simulink model "b6_goto_target"  (R2021b)
settings: Solver=VariableStepAuto  StartTime=0.0  StopTime=inf  FixedStep=0.0001  RelTol=1e-3
PreLoadFcn:
  | % Simulation parameters
  | %load exampleMap
  | 
  | % Lidar parameters
  | sensorOffset = [0,0];
  | scanAngles = linspace(-pi/3,pi/3,20)';%y = linspace(x1,x2,n) 生成 n 个点。这些点的间距为 (x2-x1)/(n-1)。
  | maxRange = 0.4;
InitFcn:
  | sampleTime = 0.05;
  | nMedianSize=3;
  |  %load boundaryMap
  | 
  | % Robot parameters
  | wheelRadius = 0.0303;
  | robotRadius = 0.06;   %小车在仿真中显示的圆形的半径大小
  | Trackwidth = 0.0847;  %定义向量场直方图算法中小车的宽度
  | 
  | % Lidar parameters
  | sensorOffset = [0,0];
  | scanAngles = linspace(-pi/3,pi/3,20)';%y = linspace(x1,x2,n) 生成 n 个点。这些点的间距为 (x2-x1)/(n-1)。
  | maxRange = 0.4;
  | 
  | %%%%%%
  | ks=1;
  | 
  | 
  | A=0.5;
  | C=1.5;
  | B=(A+C)/2;
  | 
  | wp1=[A,A; B,A;  C,A; C,B;C,C; B,C; A,C;A,B];
  | bainjie2=[-0.5,-0.5;2.5,-0.5;-0.5,2.5;2.5,2.5;]
  | WAY_P=[wp1;wp1;wp1;wp1];
  | Target=[wp1;bainjie2];
  | 
  | %%%%%%%%%%%%%%%%%%%%%%%%%%%%%%%%%%%%%%%
  | Target_robot_4=[A  A]
  | Target_robot_5=[B  A]
  | Target_robot_6=[C  A]
  | 
  | Target_robot_1=[C  C]
  | Target_robot_2=[B  C]
  | Target_robot_3=[A  C]
  | 
  | 
  | %%%%%%%%%%%%%%%%%%%%%%%%%%%%%%%%%%%%
  | 
  | 
  | init_pose_1=[A    A  pi/2]';
  | init_pose_2=[B    A  pi/2]';
  | init_pose_3=[C    A  pi/2]';
  | init_pose_4=[C    C  -pi/2]';
  | init_pose_5=[B    C  -pi/2]';
  | init_pose_6=[A    C  -pi/2]';
  | 
  | 
  | 
  | 
  | %{
  | %初始位置 交叉
  | 
  | init_pose_1=[C    C    0]';
  | init_pose_2=[B    C    0]';
  | init_pose_3=[A    C  0]';
  | init_pose_4=[A    A  0]';
  | init_pose_5=[B    A  0]';
  | init_pose_6=[C    A  0]';
  | 
  | 
  | 
  | 
  | 
  | %初始位置
  | 
  | init_pose_1=[1    1    0]';
  | init_pose_2=[1.8  1    0]';
  | init_pose_3=[0.4  1.8  0]';
  | init_pose_4=[1.6  1.6  0]';
  | init_pose_5=[0.4  0.8  0]';
  | init_pose_6=[0.8  0.6  0]';
  | %}
  | 
  | 
  | % paremeters of pure persuit
  | desired_v=0.2
  | desired_w=10
  | desired_lookahead=0.1
  | 
  | % paremeters of recovery
  | %recovery_w=0.5
  | recovery_w=2
undefined symbols (not defined in the file or in its folder): Angular, DiscIntNeverNeededParam, Linear, Pose, Twist
libraries: robotlib x45, dspstat3 x18, mobileRoboticsLib x13, robotalgslib x12, robotmobilelib x6
(part 1 of 4)
settings Model: SimulationMode=accelerator  Creator=scastro  LastModifiedBy=FCS
settings SolverCC: AlgebraicLoopSolver=TrustRegion
settings DataIOCC: ReturnWorkspaceOutputs=off
settings OptimizationCC: EnhancedBackFolding=on  PassReuseOutputArgsAs=Individual arguments  ZeroExternalMemoryAtStartup=off  ZeroInternalMemoryAtStartup=off  MaxStackSize=64  OptimizeBlockOrder=speed  DifferentSizesBufferReuse=on  OptimizationCustomize=off  EfficientTunableParamExpr=on
settings DebuggingCC: ParameterTunabilityLossMsg=error  PregeneratedLibrarySubsystemCodeDiagnostic=none  SFMachineParentedDataDiag=warning  ArithmeticOperatorsInVariantConditions=warning
settings HardwareCC: ProdBitPerPointer=32  ProdBitPerSizeT=32  ProdBitPerPtrDiffT=32  ProdLargestAtomicFloat=None  ProdIntDivRoundTo=Undefined  ProdEndianess=Unspecified  ProdWordSize=32  ProdHWDeviceType=Generic->Unspecified (assume 32-bit Generic)
settings SFSimCC: SimUseLocalCustomCode=off  CustomCodeUndefinedFunction=UseInterfaceOnly
settings RTWCC: Description=Embedded Coder  SystemTargetFile=ert.tlc  HardwareBoard=Robot Operating System (ROS)  TLCOptions="-aInlineSetEventsForThisBaseRateFcn=TLC_FALSE -aSuppressMultiTaskScheduler=TLC_FALSE  -aRateBasedStepFcn=0"  TemplateMakefile=ert_default_tmf  RTWUseLocalCustomCode=off  Toolchain=Catkin  TargetLang=C++
settings CodeAppCC: ForceParamTrailComments=on  IgnoreCustomStorageClasses=off  OperatorAnnotations=on  SimulinkDataObjDesc=on  SFDataObjDesc=on  InsertBlockDesc=on

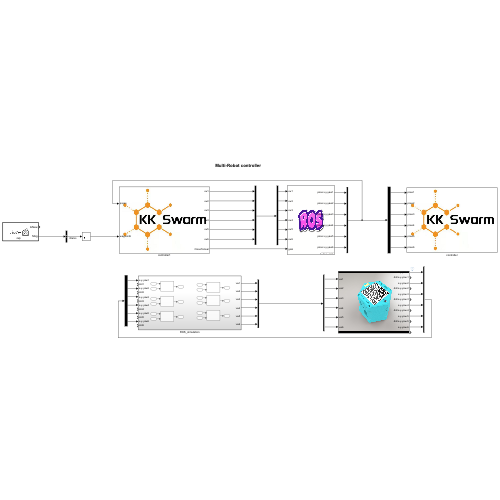
[thumbnail: Simulink's stored preview of the top-level diagram]
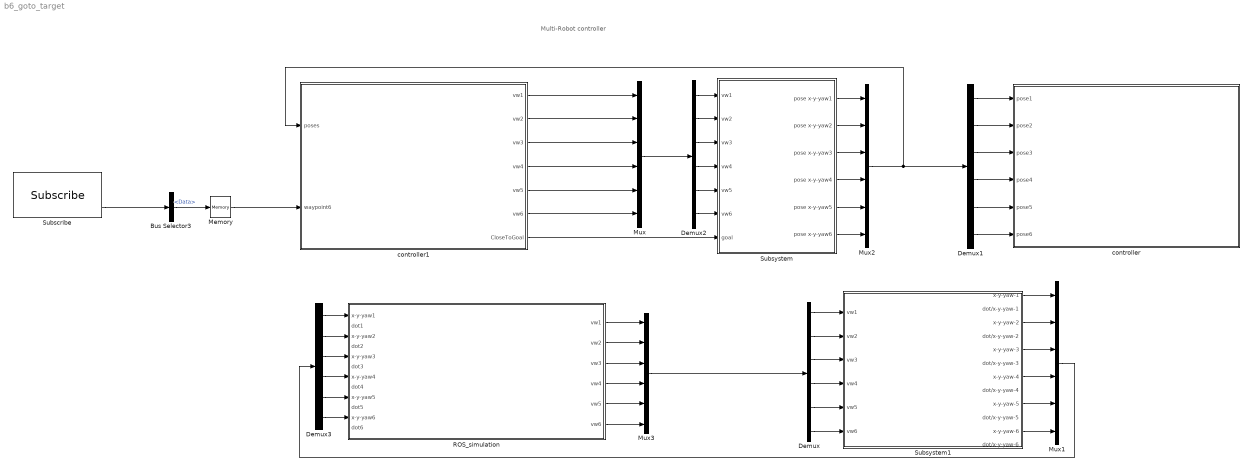
== system b6_goto_target ==
  note: Multi-Robot controller
  Bus Selector3 : BusSelector  OutputSignals=Data
  Demux{,1..3} (4 alike) : Demux  Outputs=6
  Memory : Memory  InitialCondition=123567
  Mux{,1..3} (4 alike) : Mux  Inputs=6
  ROS_simulation : Subsystem
  Subscribe : robotlib/Subscribe  topicSource=Select from ROS network  topic=/wp  messageType=std_msgs/Float64  SampleTime=-1  legacyBusStruct=off  messageQueueLength=51
  Subsystem : Subsystem
      mask Display: image('$imagefile'); % 使用工具条上的 "编辑图像" 进行更改。
  Subsystem1 : Subsystem
      mask Display: image('$imagefile'); % 使用工具条上的 "编辑图像" 进行更改。
  controller : Subsystem
      mask Display: image('$imagefile'); % 使用工具条上的 "编辑图像" 进行更改。
  controller1 : Subsystem
      mask Display: image('$imagefile'); % 使用工具条上的 "编辑图像" 进行更改。
  wires:
  Subsystem1/1(x-y-yaw-1) -> Mux1/1
  Subsystem1/3(x-y-yaw-2) -> Mux1/2
  Demux/1 -> Subsystem1/1(vw1)
  Demux/2 -> Subsystem1/2(vw2)
  Subsystem1/5(x-y-yaw-3) -> Mux1/3
  Subsystem1/7(x-y-yaw-4) -> Mux1/4
  Subsystem1/9(x-y-yaw-5) -> Mux1/5
  Subsystem1/11(x-y-yaw-6) -> Mux1/6
  Demux/3 -> Subsystem1/3(vw3)
  Demux/4 -> Subsystem1/4(vw4)
  Demux/5 -> Subsystem1/5(vw5)
  Demux/6 -> Subsystem1/6(vw6)
  ROS_simulation/1(vw1) -> Mux3/1
  ROS_simulation/2(vw2) -> Mux3/2
  ROS_simulation/4(vw4) -> Mux3/4
  ROS_simulation/5(vw5) -> Mux3/5
  ROS_simulation/6(vw6) -> Mux3/6
  ROS_simulation/3(vw3) -> Mux3/3
  Demux3/1 -> ROS_simulation/1(x-y-yaw1)
  Demux3/2 -> ROS_simulation/3(x-y-yaw2)
  Demux3/6 -> ROS_simulation/11(x-y-yaw6)
  Demux3/5 -> ROS_simulation/9(x-y-yaw5)
  Demux3/4 -> ROS_simulation/7(x-y-yaw4)
  Demux3/3 -> ROS_simulation/5(x-y-yaw3)
  Mux3/1 -> Demux/1
  Mux1/1 -> Demux3/1
  Demux1/1 -> controller/1(pose1)
  Demux1/4 -> controller/4(pose4)
  Mux/1 -> Demux2/1
  Subsystem/5(pose x-y-yaw5) -> Mux2/5
  Subsystem/3(pose x-y-yaw3) -> Mux2/3
  Subsystem/1(pose x-y-yaw1) -> Mux2/1
  Demux1/2 -> controller/2(pose2)
  Subsystem/6(pose x-y-yaw6) -> Mux2/6
  Demux2/3 -> Subsystem/3(vw3)
  Memory/1 -> controller1/2(waypoint6)
  Bus Selector3/1 -> Memory/1  "<Data>"
  Demux2/5 -> Subsystem/5(vw5)
  Demux2/2 -> Subsystem/2(vw2)
  Demux1/3 -> controller/3(pose3)
  Subsystem/2(pose x-y-yaw2) -> Mux2/2
  Mux2/1 -> controller1/1(poses), Demux1/1
  Demux2/6 -> Subsystem/6(vw6)
  Subsystem/4(pose x-y-yaw4) -> Mux2/4
  Demux1/6 -> controller/6(pose6)
  Demux2/1 -> Subsystem/1(vw1)
  Demux1/5 -> controller/5(pose5)
  Subscribe/2 -> Bus Selector3/1
  Demux2/4 -> Subsystem/4(vw4)
  controller1/7(CloseToGoal) -> Subsystem/7(goal)
  controller1/1(vw1) -> Mux/1
  controller1/2(vw2) -> Mux/2
  controller1/3(vw3) -> Mux/3
  controller1/4(vw4) -> Mux/4
  controller1/5(vw5) -> Mux/5
  controller1/6(vw6) -> Mux/6

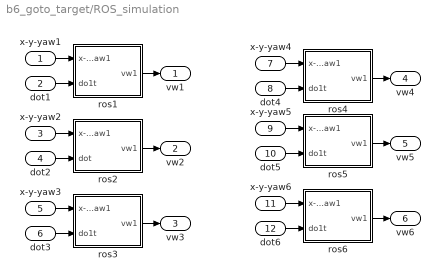
== system b6_goto_target/ROS_simulation ==
  x-y-yaw1 : Inport
  dot1 : Inport  Port=2
  x-y-yaw2 : Inport  Port=3
  dot2 : Inport  Port=4
  x-y-yaw3 : Inport  Port=5
  dot3 : Inport  Port=6
  x-y-yaw4 : Inport  Port=7
  dot4 : Inport  Port=8
  x-y-yaw5 : Inport  Port=9
  dot5 : Inport  Port=10
  x-y-yaw6 : Inport  Port=11
  dot6 : Inport  Port=12
  ros1 : Subsystem
  ros2 : Subsystem
  ros3 : Subsystem
  ros4 : Subsystem
  ros5 : Subsystem
  ros6 : Subsystem
  vw1 : Outport
  vw2 : Outport  Port=2
  vw3 : Outport  Port=3
  vw4 : Outport  Port=4
  vw5 : Outport  Port=5
  vw6 : Outport  Port=6
  wires:
  ros5/1(vw1) -> vw5/1
  ros2/1(vw1) -> vw2/1
  dot3/1 -> ros3/2(do1t)
  x-y-yaw5/1 -> ros5/1(x-y-yaw1)
  ros3/1(vw1) -> vw3/1
  dot2/1 -> ros2/2(dot)
  x-y-yaw2/1 -> ros2/1(x-y-yaw1)
  dot5/1 -> ros5/2(do1t)
  dot4/1 -> ros4/2(do1t)
  x-y-yaw4/1 -> ros4/1(x-y-yaw1)
  ros4/1(vw1) -> vw4/1
  x-y-yaw3/1 -> ros3/1(x-y-yaw1)
  dot6/1 -> ros6/2(do1t)
  x-y-yaw6/1 -> ros6/1(x-y-yaw1)
  dot1/1 -> ros1/2(do1t)
  ros6/1(vw1) -> vw6/1
  x-y-yaw1/1 -> ros1/1(x-y-yaw1)
  ros1/1(vw1) -> vw1/1

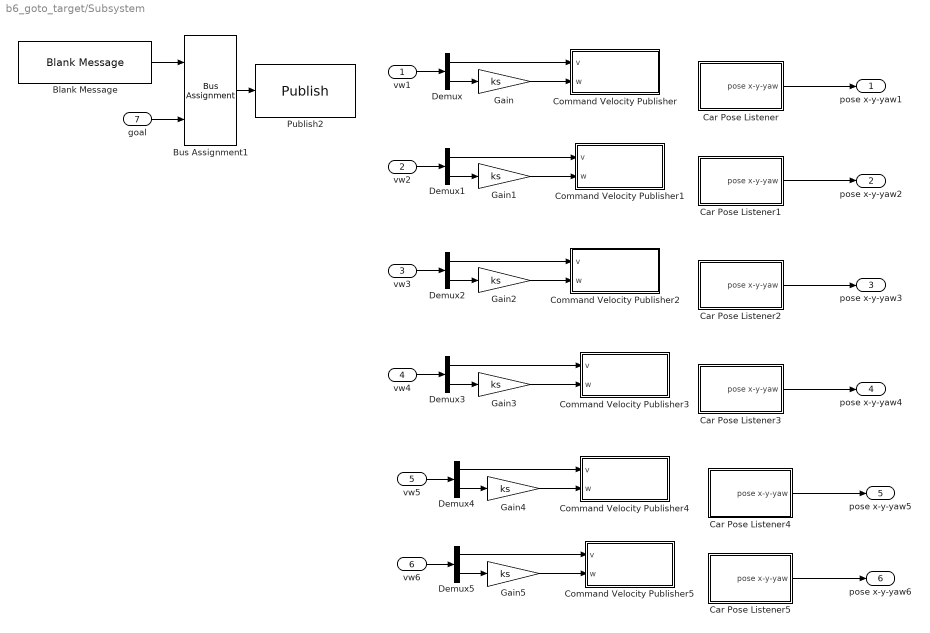
== system b6_goto_target/Subsystem ==
  vw1 : Inport
  vw2 : Inport  Port=2
  vw3 : Inport  Port=3
  vw4 : Inport  Port=4
  vw5 : Inport  Port=5
  vw6 : Inport  Port=6
  goal : Inport  Port=7
  Blank Message : robotlib/Blank Message  messageClass=Message  entityType=std_msgs/Float64  messageType=std_msgs/Float64  SampleTime=inf  legacyBusStruct=off
  Bus Assignment1 : BusAssignment  DialogController=Simulink.DDGSource_BusAssignment  AssignedSignals=Data
  Car Pose Listener : Subsystem
  Car Pose Listener1 : Subsystem
  Car Pose Listener2 : Subsystem
  Car Pose Listener3 : Subsystem
  Car Pose Listener4 : Subsystem
  Car Pose Listener5 : Subsystem
  Command Velocity Publisher : Subsystem
  Command Velocity Publisher1 : Subsystem
  Command Velocity Publisher2 : Subsystem
  Command Velocity Publisher3 : Subsystem
  Command Velocity Publisher4 : Subsystem
  Command Velocity Publisher5 : Subsystem
  Demux{,1..5} (6 alike) : Demux  Outputs=2
  Gain{,1..5} (6 alike) : Gain  Gain=ks
  Publish2 : robotlib/Publish  topicSource=Specify your own  topic=/close_goal  messageType=std_msgs/Float64  legacyBusStruct=off  messageQueueLength=105
  pose x-y-yaw1 : Outport
  pose x-y-yaw2 : Outport  Port=2
  pose x-y-yaw3 : Outport  Port=3
  pose x-y-yaw4 : Outport  Port=4
  pose x-y-yaw5 : Outport  Port=5
  pose x-y-yaw6 : Outport  Port=6
  wires:
  Gain/1 -> Command Velocity Publisher/2(w)
  Demux/2 -> Gain/1
  Car Pose Listener/1(pose x-y-yaw) -> pose x-y-yaw1/1
  Demux/1 -> Command Velocity Publisher/1(v)
  vw1/1 -> Demux/1
  Car Pose Listener1/1(pose x-y-yaw) -> pose x-y-yaw2/1
  Gain1/1 -> Command Velocity Publisher1/2(w)
  vw2/1 -> Demux1/1
  Demux1/2 -> Gain1/1
  Demux1/1 -> Command Velocity Publisher1/1(v)
  Car Pose Listener2/1(pose x-y-yaw) -> pose x-y-yaw3/1
  Gain2/1 -> Command Velocity Publisher2/2(w)
  vw3/1 -> Demux2/1
  Demux2/2 -> Gain2/1
  Demux2/1 -> Command Velocity Publisher2/1(v)
  Car Pose Listener3/1(pose x-y-yaw) -> pose x-y-yaw4/1
  Gain3/1 -> Command Velocity Publisher3/2(w)
  vw4/1 -> Demux3/1
  Demux3/2 -> Gain3/1
  Demux3/1 -> Command Velocity Publisher3/1(v)
  Car Pose Listener4/1(pose x-y-yaw) -> pose x-y-yaw5/1
  Gain4/1 -> Command Velocity Publisher4/2(w)
  vw5/1 -> Demux4/1
  Demux4/2 -> Gain4/1
  Car Pose Listener5/1(pose x-y-yaw) -> pose x-y-yaw6/1
  Gain5/1 -> Command Velocity Publisher5/2(w)
  vw6/1 -> Demux5/1
  Demux5/2 -> Gain5/1
  Demux5/1 -> Command Velocity Publisher5/1(v)
  Bus Assignment1/1 -> Publish2/1
  Blank Message/1 -> Bus Assignment1/1
  goal/1 -> Bus Assignment1/2
  Demux4/1 -> Command Velocity Publisher4/1(v)

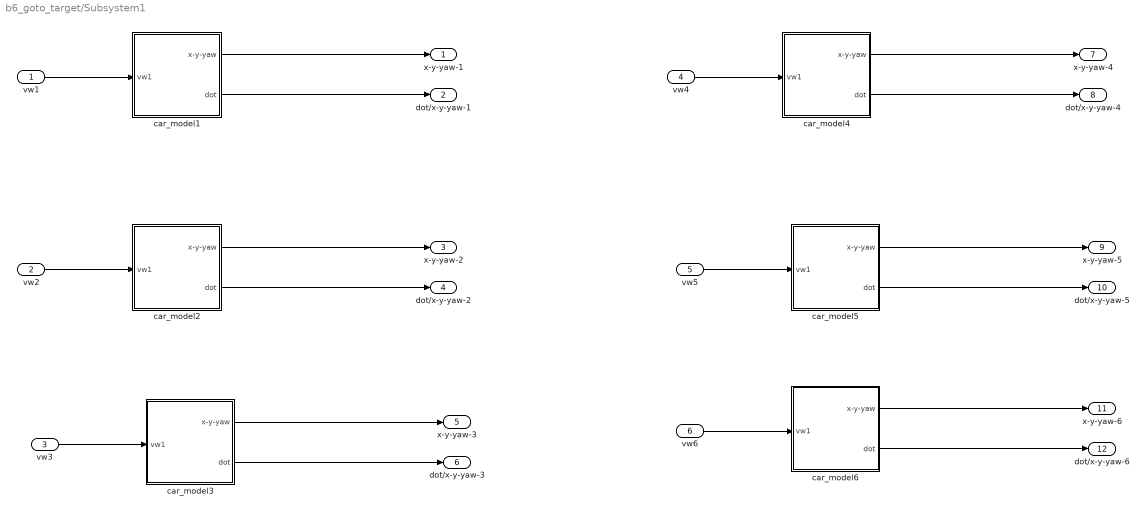
== system b6_goto_target/Subsystem1 ==
  vw1 : Inport
  vw2 : Inport  Port=2
  vw3 : Inport  Port=3
  vw4 : Inport  Port=4
  vw5 : Inport  Port=5
  vw6 : Inport  Port=6
  car_model1 : Subsystem
  car_model2 : Subsystem
  car_model3 : Subsystem
  car_model4 : Subsystem
  car_model5 : Subsystem
  car_model6 : Subsystem
  x-y-yaw-1 : Outport
  dot/x-y-yaw-1 : Outport  Port=2
  x-y-yaw-2 : Outport  Port=3
  dot/x-y-yaw-2 : Outport  Port=4
  x-y-yaw-3 : Outport  Port=5
  dot/x-y-yaw-3 : Outport  Port=6
  x-y-yaw-4 : Outport  Port=7
  dot/x-y-yaw-4 : Outport  Port=8
  x-y-yaw-5 : Outport  Port=9
  dot/x-y-yaw-5 : Outport  Port=10
  x-y-yaw-6 : Outport  Port=11
  dot/x-y-yaw-6 : Outport  Port=12
  wires:
  car_model1/1(x-y-yaw) -> x-y-yaw-1/1
  vw1/1 -> car_model1/1(vw1)
  car_model1/2(dot) -> dot/x-y-yaw-1/1
  car_model2/2(dot) -> dot/x-y-yaw-2/1
  vw2/1 -> car_model2/1(vw1)
  car_model2/1(x-y-yaw) -> x-y-yaw-2/1
  car_model3/1(x-y-yaw) -> x-y-yaw-3/1
  vw3/1 -> car_model3/1(vw1)
  car_model3/2(dot) -> dot/x-y-yaw-3/1
  car_model4/1(x-y-yaw) -> x-y-yaw-4/1
  vw4/1 -> car_model4/1(vw1)
  car_model4/2(dot) -> dot/x-y-yaw-4/1
  car_model5/1(x-y-yaw) -> x-y-yaw-5/1
  vw5/1 -> car_model5/1(vw1)
  car_model5/2(dot) -> dot/x-y-yaw-5/1
  car_model6/1(x-y-yaw) -> x-y-yaw-6/1
  vw6/1 -> car_model6/1(vw1)
  car_model6/2(dot) -> dot/x-y-yaw-6/1

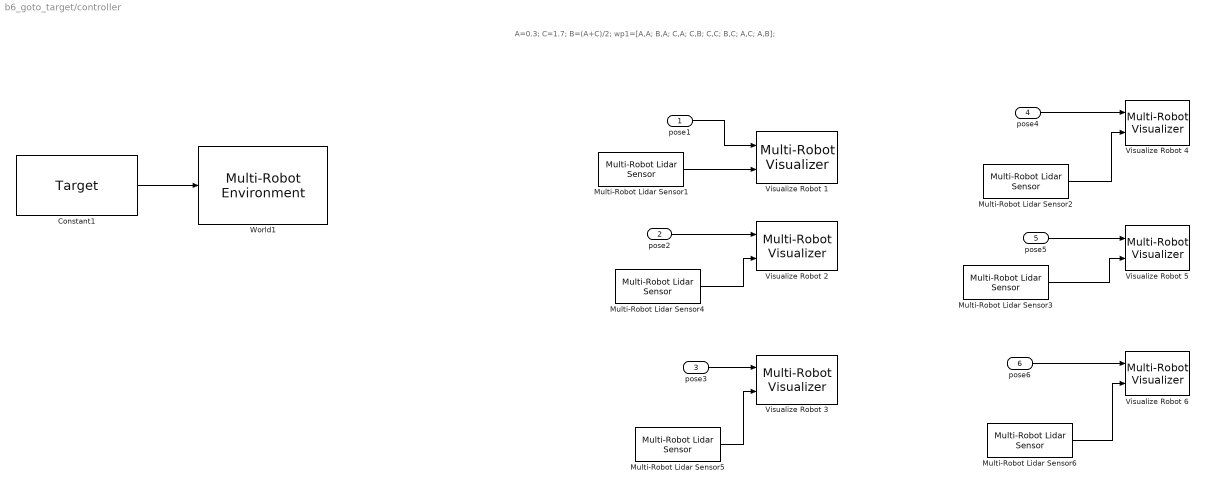
== system b6_goto_target/controller ==
  note: A=0.3;
      | C=1.7;
      | B=(A+C)/2;
      |
      | wp1=[A,A; B,A; C,A;
      | C,B;
      | C,C; B,C; A,C;
      | A,B];
  pose1 : Inport
  pose2 : Inport  Port=2
  pose3 : Inport  Port=3
  pose4 : Inport  Port=4
  pose5 : Inport  Port=5
  pose6 : Inport  Port=6
  Constant1 : Constant  Value=Target
  Multi-Robot Lidar Sensor1 : mobileRoboticsLib/Environments/Multi-Robot Lidar Sensor  robotIdx=1  sensorOffset=sensorOffset  scanAngles=scanAngles  maxRange=maxRange
      settings: SourceProductName=Mobile Robotics Simulation Toolbox
  Multi-Robot Lidar Sensor2 : mobileRoboticsLib/Environments/Multi-Robot Lidar Sensor  robotIdx=4  sensorOffset=sensorOffset  scanAngles=scanAngles  maxRange=maxRange
      settings: SourceProductName=Mobile Robotics Simulation Toolbox
  Multi-Robot Lidar Sensor3 : mobileRoboticsLib/Environments/Multi-Robot Lidar Sensor  robotIdx=5  sensorOffset=sensorOffset  scanAngles=scanAngles  maxRange=maxRange
      settings: SourceProductName=Mobile Robotics Simulation Toolbox
  Multi-Robot Lidar Sensor4 : mobileRoboticsLib/Environments/Multi-Robot Lidar Sensor  robotIdx=2  sensorOffset=sensorOffset  scanAngles=scanAngles  maxRange=maxRange
      settings: SourceProductName=Mobile Robotics Simulation Toolbox
  Multi-Robot Lidar Sensor5 : mobileRoboticsLib/Environments/Multi-Robot Lidar Sensor  robotIdx=3  sensorOffset=sensorOffset  scanAngles=scanAngles  maxRange=maxRange
      settings: SourceProductName=Mobile Robotics Simulation Toolbox
  Multi-Robot Lidar Sensor6 : mobileRoboticsLib/Environments/Multi-Robot Lidar Sensor  robotIdx=6  sensorOffset=sensorOffset  scanAngles=scanAngles  maxRange=maxRange
      settings: SourceProductName=Mobile Robotics Simulation Toolbox
  Visualize Robot 1 : mobileRoboticsLib/Environments/Multi-Robot Visualizer  idx=1  radius=robotRadius  robotColor=[0 0 1]  showTraj=off  hasLidar=on  sensorOffset=sensorOffset  scanAngles=scanAngles  maxNumScans=0  hasObjDetector=off  objDetectorOffset=[0,0]  objDetectorAngle=0  objDetectorFOV=pi/2  objDetectorMaxRange=5  hasRobotDetector=off  robotDetectorOffset=[0,0]  robotDetectorAngle=0  robotDetectorFOV=pi/3  robotDetectorMaxRange=5  robotDetectorNumDetections=0
      settings: SourceProductName=Mobile Robotics Simulation Toolbox
  Visualize Robot 2 : mobileRoboticsLib/Environments/Multi-Robot Visualizer  idx=2  radius=robotRadius  robotColor=[0 1 0]  showTraj=on  hasLidar=on  sensorOffset=sensorOffset  scanAngles=scanAngles  maxNumScans=0  hasObjDetector=off  objDetectorOffset=[0,0]  objDetectorAngle=0  objDetectorFOV=pi/2  objDetectorMaxRange=5  hasRobotDetector=off  robotDetectorOffset=[0,0]  robotDetectorAngle=0  robotDetectorFOV=pi/3  robotDetectorMaxRange=5  robotDetectorNumDetections=0
      settings: SourceProductName=Mobile Robotics Simulation Toolbox
  Visualize Robot 3 : mobileRoboticsLib/Environments/Multi-Robot Visualizer  idx=3  radius=robotRadius  robotColor=[0 1 0]  showTraj=off  hasLidar=on  sensorOffset=sensorOffset  scanAngles=scanAngles  maxNumScans=0  hasObjDetector=off  objDetectorOffset=[0,0]  objDetectorAngle=0  objDetectorFOV=pi/2  objDetectorMaxRange=5  hasRobotDetector=off  robotDetectorOffset=[0,0]  robotDetectorAngle=0  robotDetectorFOV=pi/3  robotDetectorMaxRange=5  robotDetectorNumDetections=0
      settings: SourceProductName=Mobile Robotics Simulation Toolbox
  Visualize Robot 4 : mobileRoboticsLib/Environments/Multi-Robot Visualizer  idx=4  radius=robotRadius  robotColor=[1 0 0]  showTraj=on  hasLidar=on  sensorOffset=sensorOffset  scanAngles=scanAngles  maxNumScans=0  hasObjDetector=off  objDetectorOffset=[0,0]  objDetectorAngle=0  objDetectorFOV=pi/2  objDetectorMaxRange=5  hasRobotDetector=off  robotDetectorOffset=[0,0]  robotDetectorAngle=0  robotDetectorFOV=pi/3  robotDetectorMaxRange=5  robotDetectorNumDetections=0
      settings: SourceProductName=Mobile Robotics Simulation Toolbox
  Visualize Robot 5 : mobileRoboticsLib/Environments/Multi-Robot Visualizer  idx=5  radius=robotRadius  robotColor=[1 0 1]  showTraj=off  hasLidar=on  sensorOffset=sensorOffset  scanAngles=scanAngles  maxNumScans=0  hasObjDetector=off  objDetectorOffset=[0,0]  objDetectorAngle=0  objDetectorFOV=pi/2  objDetectorMaxRange=5  hasRobotDetector=off  robotDetectorOffset=[0,0]  robotDetectorAngle=0  robotDetectorFOV=pi/3  robotDetectorMaxRange=5  robotDetectorNumDetections=0
      settings: SourceProductName=Mobile Robotics Simulation Toolbox
  Visualize Robot 6 : mobileRoboticsLib/Environments/Multi-Robot Visualizer  idx=6  radius=robotRadius  robotColor=[1 0 0]  showTraj=off  hasLidar=on  sensorOffset=sensorOffset  scanAngles=scanAngles  maxNumScans=0  hasObjDetector=off  objDetectorOffset=[0,0]  objDetectorAngle=0  objDetectorFOV=pi/2  objDetectorMaxRange=5  hasRobotDetector=off  robotDetectorOffset=[0,0]  robotDetectorAngle=0  robotDetectorFOV=pi/3  robotDetectorMaxRange=5  robotDetectorNumDetections=0
      settings: SourceProductName=Mobile Robotics Simulation Toolbox
  World1 : mobileRoboticsLib/Environments/Multi-Robot Environment  numRobots=6  showWaypoints=on  showObjects=off  objectColors=[1 0 0;0 1 0;0 0 1]  objectMarkers='s'  showRobotIds=on  plotSensorLines=on
      settings: SourceProductName=Mobile Robotics Simulation Toolbox
  wires:
  Multi-Robot Lidar Sensor5/1 -> Visualize Robot 3/2
  Multi-Robot Lidar Sensor4/1 -> Visualize Robot 2/2
  Constant1/1 -> World1/1
  pose2/1 -> Visualize Robot 2/1
  Multi-Robot Lidar Sensor1/1 -> Visualize Robot 1/2
  Multi-Robot Lidar Sensor6/1 -> Visualize Robot 6/2
  pose5/1 -> Visualize Robot 5/1
  pose3/1 -> Visualize Robot 3/1
  Multi-Robot Lidar Sensor2/1 -> Visualize Robot 4/2
  Multi-Robot Lidar Sensor3/1 -> Visualize Robot 5/2
  pose6/1 -> Visualize Robot 6/1
  pose1/1 -> Visualize Robot 1/1
  pose4/1 -> Visualize Robot 4/1

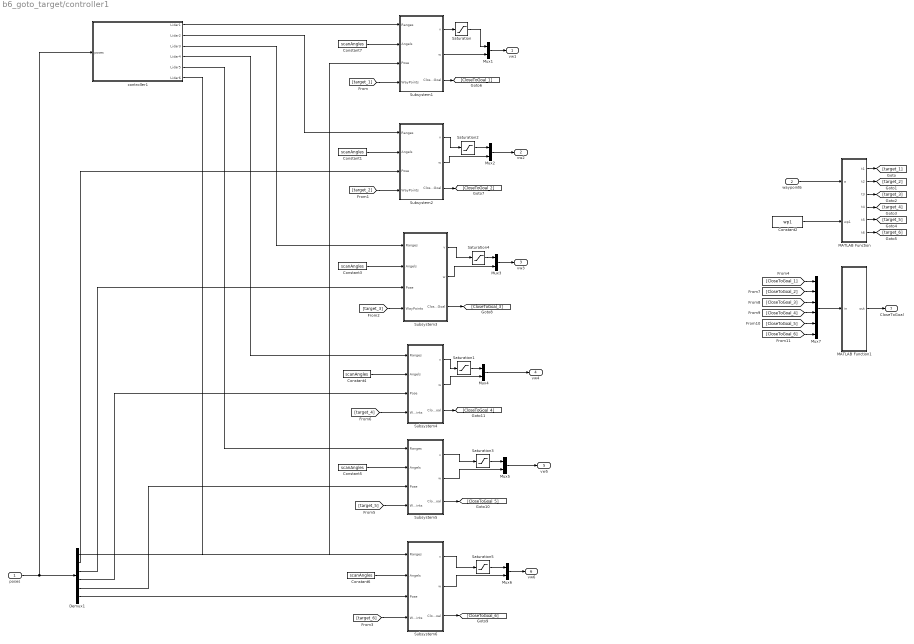
== system b6_goto_target/controller1 ==
  poses : Inport
  waypoint6 : Inport  Port=2
  Constant{1,3..7} (6 alike) : Constant  Value=scanAngles
  Constant2 : Constant  Value=wp1
  Demux1 : Demux  Outputs=6
  MATLAB Function : MATLAB Function  TreatAsAtomicUnit=on
  MATLAB Function1 : MATLAB Function  TreatAsAtomicUnit=on
  Mux{1..6} (6 alike) : Mux  Inputs=2
  Mux7 : Mux  Inputs=6
  Saturation{,1..5} (6 alike) : Saturate  UpperLimit=1  LowerLimit=0
  Subsystem1 : Subsystem
  Subsystem2 : Subsystem
  Subsystem3 : Subsystem
  Subsystem4 : Subsystem
  Subsystem5 : Subsystem
  Subsystem6 : Subsystem
  controller1 : Subsystem
      mask Display: image('$imagefile'); % 使用工具条上的 "编辑图像" 进行更改。
  vw1 : Outport
  vw2 : Outport  Port=2
  vw3 : Outport  Port=3
  vw4 : Outport  Port=4
  vw5 : Outport  Port=5
  vw6 : Outport  Port=6
  CloseToGoal : Outport  Port=7
  wires:
  poses/1 -> Demux1/1, controller1/1(poses)
  Mux1/1 -> vw1/1
  Subsystem1/1(v) -> Saturation/1
  Subsystem1/2(w) -> Mux1/2
  Subsystem1/3(CloseToGoal) -> [CloseToGoal_1]
  Saturation/1 -> Mux1/1
  MATLAB Function/4(t4) -> [target_4]
  MATLAB Function/2(t2) -> [target_2]
  MATLAB Function/5(t5) -> [target_5]
  MATLAB Function/3(t3) -> [target_3]
  MATLAB Function/1(t1) -> [target_1]
  MATLAB Function/6(t6) -> [target_6]
  waypoint6/1 -> MATLAB Function/1(a)
  Constant2/1 -> MATLAB Function/2(wp1)
  Subsystem2/3(CloseToGoal) -> [CloseToGoal_2]
  Mux2/1 -> vw2/1
  Saturation2/1 -> Mux2/1
  Subsystem2/1(v) -> Saturation2/1
  Subsystem2/2(w) -> Mux2/2
  Subsystem3/3(CloseToGoal) -> [CloseToGoal_3]
  Subsystem3/2(w) -> Mux3/2
  Subsystem3/1(v) -> Saturation4/1
  Mux3/1 -> vw3/1
  Saturation4/1 -> Mux3/1
  Subsystem4/2(w) -> Mux4/2
  Mux4/1 -> vw4/1
  Subsystem4/1(v) -> Saturation1/1
  Saturation1/1 -> Mux4/1
  Subsystem4/3(CloseToGoal) -> [CloseToGoal_4]
  Subsystem5/1(v) -> Saturation3/1
  Saturation3/1 -> Mux5/1
  Subsystem5/2(w) -> Mux5/2
  Subsystem5/3(CloseToGoal) -> [CloseToGoal_5]
  Mux5/1 -> vw5/1
  Saturation5/1 -> Mux6/1
  Mux6/1 -> vw6/1
  Subsystem6/2(w) -> Mux6/2
  Subsystem6/3(CloseToGoal) -> [CloseToGoal_6]
  Subsystem6/1(v) -> Saturation5/1
  [CloseToGoal_5] -> Mux7/5
  Mux7/1 -> MATLAB Function1/1(in)
  [CloseToGoal_6] -> Mux7/6
  [CloseToGoal_2] -> Mux7/2
  [CloseToGoal_4] -> Mux7/4
  [CloseToGoal_3] -> Mux7/3
  MATLAB Function1/1(out) -> CloseToGoal/1
  [CloseToGoal_1] -> Mux7/1
  Constant7/1 -> Subsystem1/2(Angels)
  Constant1/1 -> Subsystem2/2(Angels)
  Constant3/1 -> Subsystem3/2(Angels)
  Constant4/1 -> Subsystem4/2(Angels)
  Constant5/1 -> Subsystem5/2(Angels)
  Constant6/1 -> Subsystem6/2(Angels)
  controller1/1(Lidar1) -> Subsystem1/1(Ranges)
  Demux1/1 -> Subsystem1/3(Pose)
  controller1/2(Lidar2) -> Subsystem2/1(Ranges)
  Demux1/2 -> Subsystem2/3(Pose)
  controller1/3(Lidar3) -> Subsystem3/1(Ranges)
  Demux1/3 -> Subsystem3/3(Pose)
  [target_1] -> Subsystem1/4(WayPoints)
  [target_2] -> Subsystem2/4(WayPoints)
  [target_3] -> Subsystem3/4(WayPoints)
  [target_4] -> Subsystem4/4(WayPoints)
  [target_5] -> Subsystem5/4(WayPoints)
  [target_6] -> Subsystem6/4(WayPoints)
  controller1/4(Lidar4) -> Subsystem4/1(Ranges)
  controller1/5(Lidar5) -> Subsystem5/1(Ranges)
  controller1/6(Lidar6) -> Subsystem6/1(Ranges)
  Demux1/4 -> Subsystem4/3(Pose)
  Demux1/5 -> Subsystem5/3(Pose)
  Demux1/6 -> Subsystem6/3(Pose)

== system b6_goto_target/ROS_simulation/ros1 ==
  x-y-yaw1 : Inport
  do1t : Inport  Port=2
  " [x y theta]" : Demux  Outputs=3
  " [x y theta]1" : Demux  Outputs=3
  Blank Message : robotlib/Blank Message  messageClass=Message  entityType=nav_msgs/Odometry  messageType=nav_msgs/Odometry  SampleTime=inf  legacyBusStruct=off
  Bus Assignment1 : BusAssignment  DialogController=Simulink.DDGSource_BusAssignment  AssignedSignals=Pose.Pose.Position.X,Pose.Pose.Position.Y,Pose.Pose.Orientation.Z,Pose.Pose.Orientation.W,Twist.Twist.Linear.X,Twist.Twist.Linear.Y,Twist.Twist.Angular.Z
  Bus Selector3 : BusSelector  OutputSignals=Linear.X,Angular.Z
  MATLAB Function : MATLAB Function  TreatAsAtomicUnit=on
  Mux5 : Mux  Inputs=2
  Publish2 : robotlib/Publish  topicSource=Specify your own  topic=/robot_1/pose  messageType=nav_msgs/Odometry  legacyBusStruct=off  messageQueueLength=105
  Subscribe1 : robotlib/Subscribe  topicSource=Specify your own  topic=/robot_1/cmd_vel  messageType=geometry_msgs/Twist  SampleTime=-1  legacyBusStruct=off  messageQueueLength=51
  Terminator : Terminator
  Terminator1 : Terminator
  Zero-Order Hold : ZeroOrderHold  SampleTime=0.1
  Zero-Order Hold1 : ZeroOrderHold  SampleTime=0.1
  vw1 : Outport
  wires:
  " [x y theta]"/1 -> Bus Assignment1/2
  Blank Message/1 -> Bus Assignment1/1
  x-y-yaw1/1 -> Zero-Order Hold/1
  " [x y theta]"/2 -> Bus Assignment1/3
  " [x y theta]1"/2 -> Bus Assignment1/7
  " [x y theta]"/3 -> MATLAB Function/1(yaw)
  " [x y theta]1"/3 -> Bus Assignment1/8
  MATLAB Function/4(w) -> Bus Assignment1/5
  MATLAB Function/3(z) -> Bus Assignment1/4
  " [x y theta]1"/1 -> Bus Assignment1/6
  Bus Assignment1/1 -> Publish2/1
  do1t/1 -> Zero-Order Hold1/1
  MATLAB Function/1(x) -> Terminator/1
  MATLAB Function/2(y) -> Terminator1/1
  Bus Selector3/1 -> Mux5/1  "<X>"
  Bus Selector3/2 -> Mux5/2  "<Z>"
  Subscribe1/2 -> Bus Selector3/1
  Mux5/1 -> vw1/1
  Zero-Order Hold1/1 -> " [x y theta]1"/1
  Zero-Order Hold/1 -> " [x y theta]"/1

== system b6_goto_target/ROS_simulation/ros2 ==
  x-y-yaw1 : Inport
  dot : Inport  Port=2
  " [x y theta]" : Demux  Outputs=3
  " [x y theta]1" : Demux  Outputs=3
  Blank Message : robotlib/Blank Message  messageClass=Message  entityType=nav_msgs/Odometry  messageType=nav_msgs/Odometry  SampleTime=inf  legacyBusStruct=off
  Bus Assignment1 : BusAssignment  DialogController=Simulink.DDGSource_BusAssignment  AssignedSignals=Pose.Pose.Position.X,Pose.Pose.Position.Y,Pose.Pose.Orientation.Z,Pose.Pose.Orientation.W,Twist.Twist.Linear.X,Twist.Twist.Linear.Y,Twist.Twist.Angular.Z
  Bus Selector3 : BusSelector  OutputSignals=Linear.X,Angular.Z
  MATLAB Function : MATLAB Function  TreatAsAtomicUnit=on
  Mux5 : Mux  Inputs=2
  Publish2 : robotlib/Publish  topicSource=Specify your own  topic=/robot_2/pose  messageType=nav_msgs/Odometry  legacyBusStruct=off  messageQueueLength=105
  Subscribe1 : robotlib/Subscribe  topicSource=Specify your own  topic=/robot_2/cmd_vel  messageType=geometry_msgs/Twist  SampleTime=-1  legacyBusStruct=off  messageQueueLength=51
  Terminator : Terminator
  Terminator1 : Terminator
  Zero-Order Hold : ZeroOrderHold  SampleTime=0.1
  Zero-Order Hold1 : ZeroOrderHold  SampleTime=0.1
  vw1 : Outport
  wires:
  " [x y theta]"/1 -> Bus Assignment1/2
  Blank Message/1 -> Bus Assignment1/1
  x-y-yaw1/1 -> Zero-Order Hold/1
  " [x y theta]"/2 -> Bus Assignment1/3
  " [x y theta]1"/2 -> Bus Assignment1/7
  " [x y theta]"/3 -> MATLAB Function/1(yaw)
  " [x y theta]1"/3 -> Bus Assignment1/8
  MATLAB Function/4(w) -> Bus Assignment1/5
  MATLAB Function/3(z) -> Bus Assignment1/4
  " [x y theta]1"/1 -> Bus Assignment1/6
  Bus Assignment1/1 -> Publish2/1
  dot/1 -> Zero-Order Hold1/1
  MATLAB Function/1(x) -> Terminator/1
  MATLAB Function/2(y) -> Terminator1/1
  Bus Selector3/1 -> Mux5/1  "<X>"
  Bus Selector3/2 -> Mux5/2  "<Z>"
  Subscribe1/2 -> Bus Selector3/1
  Mux5/1 -> vw1/1
  Zero-Order Hold/1 -> " [x y theta]"/1
  Zero-Order Hold1/1 -> " [x y theta]1"/1

== system b6_goto_target/ROS_simulation/ros3 ==
  x-y-yaw1 : Inport
  do1t : Inport  Port=2
  " [x y theta]" : Demux  Outputs=3
  " [x y theta]1" : Demux  Outputs=3
  Blank Message : robotlib/Blank Message  messageClass=Message  entityType=nav_msgs/Odometry  messageType=nav_msgs/Odometry  SampleTime=inf  legacyBusStruct=off
  Bus Assignment1 : BusAssignment  DialogController=Simulink.DDGSource_BusAssignment  AssignedSignals=Pose.Pose.Position.X,Pose.Pose.Position.Y,Pose.Pose.Orientation.Z,Pose.Pose.Orientation.W,Twist.Twist.Linear.X,Twist.Twist.Linear.Y,Twist.Twist.Angular.Z
  Bus Selector3 : BusSelector  OutputSignals=Linear.X,Angular.Z
  MATLAB Function : MATLAB Function  TreatAsAtomicUnit=on
  Mux5 : Mux  Inputs=2
  Publish2 : robotlib/Publish  topicSource=Specify your own  topic=/robot_3/pose  messageType=nav_msgs/Odometry  legacyBusStruct=off  messageQueueLength=105
  Subscribe1 : robotlib/Subscribe  topicSource=Specify your own  topic=/robot_3/cmd_vel  messageType=geometry_msgs/Twist  SampleTime=-1  legacyBusStruct=off  messageQueueLength=51
  Terminator : Terminator
  Terminator1 : Terminator
  Zero-Order Hold : ZeroOrderHold  SampleTime=0.1
  Zero-Order Hold1 : ZeroOrderHold  SampleTime=0.1
  vw1 : Outport
  wires:
  " [x y theta]"/1 -> Bus Assignment1/2
  Blank Message/1 -> Bus Assignment1/1
  x-y-yaw1/1 -> Zero-Order Hold/1
  " [x y theta]"/2 -> Bus Assignment1/3
  " [x y theta]1"/2 -> Bus Assignment1/7
  " [x y theta]"/3 -> MATLAB Function/1(yaw)
  " [x y theta]1"/3 -> Bus Assignment1/8
  MATLAB Function/4(w) -> Bus Assignment1/5
  MATLAB Function/3(z) -> Bus Assignment1/4
  " [x y theta]1"/1 -> Bus Assignment1/6
  Bus Assignment1/1 -> Publish2/1
  do1t/1 -> Zero-Order Hold1/1
  MATLAB Function/1(x) -> Terminator/1
  MATLAB Function/2(y) -> Terminator1/1
  Bus Selector3/1 -> Mux5/1  "<X>"
  Bus Selector3/2 -> Mux5/2  "<Z>"
  Subscribe1/2 -> Bus Selector3/1
  Mux5/1 -> vw1/1
  Zero-Order Hold/1 -> " [x y theta]"/1
  Zero-Order Hold1/1 -> " [x y theta]1"/1

== system b6_goto_target/ROS_simulation/ros4 ==
  x-y-yaw1 : Inport
  do1t : Inport  Port=2
  " [x y theta]" : Demux  Outputs=3
  " [x y theta]1" : Demux  Outputs=3
  Blank Message : robotlib/Blank Message  messageClass=Message  entityType=nav_msgs/Odometry  messageType=nav_msgs/Odometry  SampleTime=inf  legacyBusStruct=off
  Bus Assignment1 : BusAssignment  DialogController=Simulink.DDGSource_BusAssignment  AssignedSignals=Pose.Pose.Position.X,Pose.Pose.Position.Y,Pose.Pose.Orientation.Z,Pose.Pose.Orientation.W,Twist.Twist.Linear.X,Twist.Twist.Linear.Y,Twist.Twist.Angular.Z
  Bus Selector3 : BusSelector  OutputSignals=Linear.X,Angular.Z
  MATLAB Function : MATLAB Function  TreatAsAtomicUnit=on
  Mux5 : Mux  Inputs=2
  Publish2 : robotlib/Publish  topicSource=Specify your own  topic=/robot_4/pose  messageType=nav_msgs/Odometry  legacyBusStruct=off  messageQueueLength=105
  Subscribe1 : robotlib/Subscribe  topicSource=Specify your own  topic=/robot_4/cmd_vel  messageType=geometry_msgs/Twist  SampleTime=-1  legacyBusStruct=off  messageQueueLength=51
  Terminator : Terminator
  Terminator1 : Terminator
  Zero-Order Hold : ZeroOrderHold  SampleTime=0.1
  Zero-Order Hold1 : ZeroOrderHold  SampleTime=0.1
  vw1 : Outport
  wires:
  " [x y theta]"/1 -> Bus Assignment1/2
  Blank Message/1 -> Bus Assignment1/1
  x-y-yaw1/1 -> Zero-Order Hold/1
  " [x y theta]"/2 -> Bus Assignment1/3
  " [x y theta]1"/2 -> Bus Assignment1/7
  " [x y theta]"/3 -> MATLAB Function/1(yaw)
  " [x y theta]1"/3 -> Bus Assignment1/8
  MATLAB Function/4(w) -> Bus Assignment1/5
  MATLAB Function/3(z) -> Bus Assignment1/4
  " [x y theta]1"/1 -> Bus Assignment1/6
  Bus Assignment1/1 -> Publish2/1
  do1t/1 -> Zero-Order Hold1/1
  MATLAB Function/1(x) -> Terminator/1
  MATLAB Function/2(y) -> Terminator1/1
  Bus Selector3/1 -> Mux5/1  "<X>"
  Bus Selector3/2 -> Mux5/2  "<Z>"
  Subscribe1/2 -> Bus Selector3/1
  Mux5/1 -> vw1/1
  Zero-Order Hold/1 -> " [x y theta]"/1
  Zero-Order Hold1/1 -> " [x y theta]1"/1

== system b6_goto_target/ROS_simulation/ros5 ==
  x-y-yaw1 : Inport
  do1t : Inport  Port=2
  " [x y theta]" : Demux  Outputs=3
  " [x y theta]1" : Demux  Outputs=3
  Blank Message : robotlib/Blank Message  messageClass=Message  entityType=nav_msgs/Odometry  messageType=nav_msgs/Odometry  SampleTime=inf  legacyBusStruct=off
  Bus Assignment1 : BusAssignment  DialogController=Simulink.DDGSource_BusAssignment  AssignedSignals=Pose.Pose.Position.X,Pose.Pose.Position.Y,Pose.Pose.Orientation.Z,Pose.Pose.Orientation.W,Twist.Twist.Linear.X,Twist.Twist.Linear.Y,Twist.Twist.Angular.Z
  Bus Selector3 : BusSelector  OutputSignals=Linear.X,Angular.Z
  MATLAB Function : MATLAB Function  TreatAsAtomicUnit=on
  Mux5 : Mux  Inputs=2
  Publish2 : robotlib/Publish  topicSource=Specify your own  topic=/robot_5/pose  messageType=nav_msgs/Odometry  legacyBusStruct=off  messageQueueLength=105
  Subscribe1 : robotlib/Subscribe  topicSource=Specify your own  topic=/robot_5/cmd_vel  messageType=geometry_msgs/Twist  SampleTime=-1  legacyBusStruct=off  messageQueueLength=51
  Terminator : Terminator
  Terminator1 : Terminator
  Zero-Order Hold : ZeroOrderHold  SampleTime=0.1
  Zero-Order Hold1 : ZeroOrderHold  SampleTime=0.1
  vw1 : Outport
  wires:
  " [x y theta]"/1 -> Bus Assignment1/2
  Blank Message/1 -> Bus Assignment1/1
  x-y-yaw1/1 -> Zero-Order Hold/1
  " [x y theta]"/2 -> Bus Assignment1/3
  " [x y theta]1"/2 -> Bus Assignment1/7
  " [x y theta]"/3 -> MATLAB Function/1(yaw)
  " [x y theta]1"/3 -> Bus Assignment1/8
  MATLAB Function/4(w) -> Bus Assignment1/5
  MATLAB Function/3(z) -> Bus Assignment1/4
  " [x y theta]1"/1 -> Bus Assignment1/6
  Bus Assignment1/1 -> Publish2/1
  do1t/1 -> Zero-Order Hold1/1
  MATLAB Function/1(x) -> Terminator/1
  MATLAB Function/2(y) -> Terminator1/1
  Bus Selector3/1 -> Mux5/1  "<X>"
  Bus Selector3/2 -> Mux5/2  "<Z>"
  Subscribe1/2 -> Bus Selector3/1
  Mux5/1 -> vw1/1
  Zero-Order Hold/1 -> " [x y theta]"/1
  Zero-Order Hold1/1 -> " [x y theta]1"/1

== system b6_goto_target/ROS_simulation/ros6 ==
  x-y-yaw1 : Inport
  do1t : Inport  Port=2
  " [x y theta]" : Demux  Outputs=3
  " [x y theta]1" : Demux  Outputs=3
  Blank Message : robotlib/Blank Message  messageClass=Message  entityType=nav_msgs/Odometry  messageType=nav_msgs/Odometry  SampleTime=inf  legacyBusStruct=off
  Bus Assignment1 : BusAssignment  DialogController=Simulink.DDGSource_BusAssignment  AssignedSignals=Pose.Pose.Position.X,Pose.Pose.Position.Y,Pose.Pose.Orientation.Z,Pose.Pose.Orientation.W,Twist.Twist.Linear.X,Twist.Twist.Linear.Y,Twist.Twist.Angular.Z
  Bus Selector3 : BusSelector  OutputSignals=Linear.X,Angular.Z
  MATLAB Function : MATLAB Function  TreatAsAtomicUnit=on
  Mux5 : Mux  Inputs=2
  Publish2 : robotlib/Publish  topicSource=Specify your own  topic=/robot_6/pose  messageType=nav_msgs/Odometry  legacyBusStruct=off  messageQueueLength=105
  Subscribe1 : robotlib/Subscribe  topicSource=Specify your own  topic=/robot_6/cmd_vel  messageType=geometry_msgs/Twist  SampleTime=-1  legacyBusStruct=off  messageQueueLength=51
  Terminator : Terminator
  Terminator1 : Terminator
  Zero-Order Hold : ZeroOrderHold  SampleTime=0.1
  Zero-Order Hold1 : ZeroOrderHold  SampleTime=0.1
  vw1 : Outport
  wires:
  " [x y theta]"/1 -> Bus Assignment1/2
  Blank Message/1 -> Bus Assignment1/1
  x-y-yaw1/1 -> Zero-Order Hold/1
  " [x y theta]"/2 -> Bus Assignment1/3
  " [x y theta]1"/2 -> Bus Assignment1/7
  " [x y theta]"/3 -> MATLAB Function/1(yaw)
  " [x y theta]1"/3 -> Bus Assignment1/8
  MATLAB Function/4(w) -> Bus Assignment1/5
  MATLAB Function/3(z) -> Bus Assignment1/4
  " [x y theta]1"/1 -> Bus Assignment1/6
  Bus Assignment1/1 -> Publish2/1
  do1t/1 -> Zero-Order Hold1/1
  MATLAB Function/1(x) -> Terminator/1
  MATLAB Function/2(y) -> Terminator1/1
  Bus Selector3/1 -> Mux5/1  "<X>"
  Bus Selector3/2 -> Mux5/2  "<Z>"
  Subscribe1/2 -> Bus Selector3/1
  Mux5/1 -> vw1/1
  Zero-Order Hold/1 -> " [x y theta]"/1
  Zero-Order Hold1/1 -> " [x y theta]1"/1

== system b6_goto_target/Subsystem/Car Pose Listener ==
  Subscribe : robotlib/Subscribe  topicSource=Specify your own  topic=/robot_1/pose  messageType=nav_msgs/Odometry  SampleTime=-1  legacyBusStruct=off  messageQueueLength=51
  Subscribe1 : robotlib/Subscribe  topicSource=Specify your own  topic=/robot_1/odometry  messageType=geometry_msgs/Twist  SampleTime=-1  legacyBusStruct=off  messageQueueLength=51
  Subsystem : Subsystem
  pose x-y-yaw : Outport
  wires:
  Subscribe/1 -> Subsystem/1(poseNew)  "IsNew"
  Subscribe/2 -> Subsystem/2(poseMsg)
  Subscribe1/1 -> Subsystem/3(VW_New)  "IsNew"
  Subscribe1/2 -> Subsystem/4(VW_Msg)
  Subsystem/1(pose) -> pose x-y-yaw/1

== system b6_goto_target/Subsystem/Car Pose Listener1 ==
  Subscribe : robotlib/Subscribe  topicSource=Specify your own  topic=/robot_2/pose  messageType=nav_msgs/Odometry  SampleTime=-1  legacyBusStruct=off  messageQueueLength=51
  Subscribe1 : robotlib/Subscribe  topicSource=Specify your own  topic=/robot_2/odometry  messageType=geometry_msgs/Twist  SampleTime=-1  legacyBusStruct=off  messageQueueLength=51
  Subsystem : Subsystem
  pose x-y-yaw : Outport
  wires:
  Subscribe/1 -> Subsystem/1(poseNew)  "IsNew"
  Subscribe/2 -> Subsystem/2(poseMsg)
  Subscribe1/2 -> Subsystem/4(VW_Msg)
  Subscribe1/1 -> Subsystem/3(VW_New)  "IsNew"
  Subsystem/1(pose) -> pose x-y-yaw/1

== system b6_goto_target/Subsystem/Car Pose Listener2 ==
  Subscribe : robotlib/Subscribe  topicSource=Specify your own  topic=/robot_3/pose  messageType=nav_msgs/Odometry  SampleTime=-1  legacyBusStruct=off  messageQueueLength=51
  Subscribe1 : robotlib/Subscribe  topicSource=Specify your own  topic=/robot_3/odometry  messageType=geometry_msgs/Twist  SampleTime=-1  legacyBusStruct=off  messageQueueLength=51
  Subsystem : Subsystem
  pose x-y-yaw : Outport
  wires:
  Subscribe/1 -> Subsystem/1(poseNew)  "IsNew"
  Subscribe/2 -> Subsystem/2(poseMsg)
  Subscribe1/1 -> Subsystem/3(VW_New)  "IsNew"
  Subscribe1/2 -> Subsystem/4(VW_Msg)
  Subsystem/1(pose) -> pose x-y-yaw/1

== system b6_goto_target/Subsystem/Car Pose Listener3 ==
  Subscribe : robotlib/Subscribe  topicSource=Specify your own  topic=/robot_4/pose  messageType=nav_msgs/Odometry  SampleTime=-1  legacyBusStruct=off  messageQueueLength=51
  Subscribe1 : robotlib/Subscribe  topicSource=Specify your own  topic=/robot_4/odometry  messageType=geometry_msgs/Twist  SampleTime=-1  legacyBusStruct=off  messageQueueLength=51
  Subsystem : Subsystem
  pose x-y-yaw : Outport
  wires:
  Subscribe/1 -> Subsystem/1(poseNew)  "IsNew"
  Subscribe/2 -> Subsystem/2(poseMsg)
  Subscribe1/1 -> Subsystem/3(VW_New)  "IsNew"
  Subscribe1/2 -> Subsystem/4(VW_Msg)
  Subsystem/1(pose) -> pose x-y-yaw/1

== system b6_goto_target/Subsystem/Car Pose Listener4 ==
  Subscribe : robotlib/Subscribe  topicSource=Specify your own  topic=/robot_5/pose  messageType=nav_msgs/Odometry  SampleTime=-1  legacyBusStruct=off  messageQueueLength=51
  Subscribe1 : robotlib/Subscribe  topicSource=Specify your own  topic=/robot_5/odometry  messageType=geometry_msgs/Twist  SampleTime=-1  legacyBusStruct=off  messageQueueLength=51
  Subsystem : Subsystem
  pose x-y-yaw : Outport
  wires:
  Subscribe/1 -> Subsystem/1(poseNew)  "IsNew"
  Subscribe/2 -> Subsystem/2(poseMsg)
  Subscribe1/1 -> Subsystem/3(VW_New)  "IsNew"
  Subscribe1/2 -> Subsystem/4(VW_Msg)
  Subsystem/1(pose) -> pose x-y-yaw/1

== system b6_goto_target/Subsystem/Car Pose Listener5 ==
  Subscribe : robotlib/Subscribe  topicSource=Specify your own  topic=/robot_6/pose  messageType=nav_msgs/Odometry  SampleTime=-1  legacyBusStruct=off  messageQueueLength=51
  Subscribe1 : robotlib/Subscribe  topicSource=Specify your own  topic=/robot_6/odometry  messageType=geometry_msgs/Twist  SampleTime=-1  legacyBusStruct=off  messageQueueLength=51
  Subsystem : Subsystem
  pose x-y-yaw : Outport
  wires:
  Subscribe/1 -> Subsystem/1(poseNew)  "IsNew"
  Subscribe/2 -> Subsystem/2(poseMsg)
  Subscribe1/1 -> Subsystem/3(VW_New)  "IsNew"
  Subscribe1/2 -> Subsystem/4(VW_Msg)
  Subsystem/1(pose) -> pose x-y-yaw/1

== system b6_goto_target/Subsystem/Command Velocity Publisher ==
  v : Inport
  w : Inport  Port=2
  Blank Message : robotlib/Blank Message  messageClass=Message  entityType=geometry_msgs/Twist  messageType=geometry_msgs/Twist  SampleTime=inf  legacyBusStruct=off
  Bus Assignment1 : BusAssignment  DialogController=Simulink.DDGSource_BusAssignment  AssignedSignals=Linear.X,Angular.Z
  Publish2 : robotlib/Publish  topicSource=Specify your own  topic=/robot_1/cmd_vel  messageType=geometry_msgs/Twist  legacyBusStruct=off  messageQueueLength=105
  wires:
  Bus Assignment1/1 -> Publish2/1
  Blank Message/1 -> Bus Assignment1/1
  v/1 -> Bus Assignment1/2
  w/1 -> Bus Assignment1/3

== system b6_goto_target/Subsystem/Command Velocity Publisher1 ==
  v : Inport
  w : Inport  Port=2
  Blank Message : robotlib/Blank Message  messageClass=Message  entityType=geometry_msgs/Twist  messageType=geometry_msgs/Twist  SampleTime=inf  legacyBusStruct=off
  Bus Assignment1 : BusAssignment  DialogController=Simulink.DDGSource_BusAssignment  AssignedSignals=Linear.X,Angular.Z
  Publish2 : robotlib/Publish  topicSource=Specify your own  topic=/robot_2/cmd_vel  messageType=geometry_msgs/Twist  legacyBusStruct=off  messageQueueLength=105
  wires:
  Bus Assignment1/1 -> Publish2/1
  Blank Message/1 -> Bus Assignment1/1
  v/1 -> Bus Assignment1/2
  w/1 -> Bus Assignment1/3

== system b6_goto_target/Subsystem/Command Velocity Publisher2 ==
  v : Inport
  w : Inport  Port=2
  Blank Message : robotlib/Blank Message  messageClass=Message  entityType=geometry_msgs/Twist  messageType=geometry_msgs/Twist  SampleTime=inf  legacyBusStruct=off
  Bus Assignment1 : BusAssignment  DialogController=Simulink.DDGSource_BusAssignment  AssignedSignals=Linear.X,Angular.Z
  Publish2 : robotlib/Publish  topicSource=Specify your own  topic=/robot_3/cmd_vel  messageType=geometry_msgs/Twist  legacyBusStruct=off  messageQueueLength=105
  wires:
  Bus Assignment1/1 -> Publish2/1
  Blank Message/1 -> Bus Assignment1/1
  v/1 -> Bus Assignment1/2
  w/1 -> Bus Assignment1/3

== system b6_goto_target/Subsystem/Command Velocity Publisher3 ==
  v : Inport
  w : Inport  Port=2
  Blank Message : robotlib/Blank Message  messageClass=Message  entityType=geometry_msgs/Twist  messageType=geometry_msgs/Twist  SampleTime=inf  legacyBusStruct=off
  Bus Assignment1 : BusAssignment  DialogController=Simulink.DDGSource_BusAssignment  AssignedSignals=Linear.X,Angular.Z
  Publish2 : robotlib/Publish  topicSource=Specify your own  topic=/robot_4/cmd_vel  messageType=geometry_msgs/Twist  legacyBusStruct=off  messageQueueLength=105
  wires:
  Bus Assignment1/1 -> Publish2/1
  Blank Message/1 -> Bus Assignment1/1
  v/1 -> Bus Assignment1/2
  w/1 -> Bus Assignment1/3

== system b6_goto_target/Subsystem/Command Velocity Publisher4 ==
  v : Inport
  w : Inport  Port=2
  Blank Message : robotlib/Blank Message  messageClass=Message  entityType=geometry_msgs/Twist  messageType=geometry_msgs/Twist  SampleTime=inf  legacyBusStruct=off
  Bus Assignment1 : BusAssignment  DialogController=Simulink.DDGSource_BusAssignment  AssignedSignals=Linear.X,Angular.Z
  Publish2 : robotlib/Publish  topicSource=Specify your own  topic=/robot_5/cmd_vel  messageType=geometry_msgs/Twist  legacyBusStruct=off  messageQueueLength=105
  wires:
  Bus Assignment1/1 -> Publish2/1
  Blank Message/1 -> Bus Assignment1/1
  v/1 -> Bus Assignment1/2
  w/1 -> Bus Assignment1/3

== system b6_goto_target/Subsystem/Command Velocity Publisher5 ==
  v : Inport
  w : Inport  Port=2
  Blank Message : robotlib/Blank Message  messageClass=Message  entityType=geometry_msgs/Twist  messageType=geometry_msgs/Twist  SampleTime=inf  legacyBusStruct=off
  Bus Assignment1 : BusAssignment  DialogController=Simulink.DDGSource_BusAssignment  AssignedSignals=Linear.X,Angular.Z
  Publish2 : robotlib/Publish  topicSource=Specify your own  topic=/robot_6/cmd_vel  messageType=geometry_msgs/Twist  legacyBusStruct=off  messageQueueLength=105
  wires:
  Bus Assignment1/1 -> Publish2/1
  Blank Message/1 -> Bus Assignment1/1
  v/1 -> Bus Assignment1/2
  w/1 -> Bus Assignment1/3

== system b6_goto_target/Subsystem1/car_model1 ==
  note: tr=0.6
      | 4T=0.6
      | 一阶系统的动态性能指标为：td=0.69T，tr=2.20T，ts=3T
  vw1 : Inport
  Demux : Demux  Outputs=2
  Differential Drive Kinematic Model1 : robotmobilelib/Differential Drive Kinematic Model  VehicleInputs=Vehicle Speed & Heading Angular Velocity  WheelRadius=0.05  WheelSpeedRange=[-inf inf]  TrackWidth=0.2  InitialState=init_pose_1  SimulateUsing=Interpreted execution
      settings: SourceProductBaseCode=RO
  Simulink顺时针为正 小车逆时针为正 : Gain  Gain=ks
  Transfer Fcn : TransferFcn  Denominator=[0.15 1]
  Transfer Fcn1 : TransferFcn  Denominator=[0.16 1]
  x-y-yaw : Outport
  dot : Outport  Port=2
  wires:
  Simulink顺时针为正 小车逆时针为正/1 -> Transfer Fcn1/1
  Transfer Fcn/1 -> Differential Drive Kinematic Model1/1
  Demux/1 -> Transfer Fcn/1
  Transfer Fcn1/1 -> Differential Drive Kinematic Model1/2
  Demux/2 -> Simulink顺时针为正 小车逆时针为正/1
  vw1/1 -> Demux/1
  Differential Drive Kinematic Model1/1 -> x-y-yaw/1
  Differential Drive Kinematic Model1/2 -> dot/1

== system b6_goto_target/Subsystem1/car_model2 ==
  note: tr=0.6
      | 4T=0.6
      | 一阶系统的动态性能指标为：td=0.69T，tr=2.20T，ts=3T
  vw1 : Inport
  Demux : Demux  Outputs=2
  Differential Drive Kinematic Model1 : robotmobilelib/Differential Drive Kinematic Model  VehicleInputs=Vehicle Speed & Heading Angular Velocity  WheelRadius=0.05  WheelSpeedRange=[-inf inf]  TrackWidth=0.2  InitialState=init_pose_2  SimulateUsing=Interpreted execution
      settings: SourceProductBaseCode=RO
  Simulink顺时针为正 小车逆时针为正 : Gain  Gain=ks
  Transfer Fcn : TransferFcn  Denominator=[0.15 1]
  Transfer Fcn1 : TransferFcn  Denominator=[0.16 1]
  x-y-yaw : Outport
  dot : Outport  Port=2
  wires:
  Simulink顺时针为正 小车逆时针为正/1 -> Transfer Fcn1/1
  Transfer Fcn/1 -> Differential Drive Kinematic Model1/1
  Demux/1 -> Transfer Fcn/1
  Transfer Fcn1/1 -> Differential Drive Kinematic Model1/2
  Demux/2 -> Simulink顺时针为正 小车逆时针为正/1
  vw1/1 -> Demux/1
  Differential Drive Kinematic Model1/1 -> x-y-yaw/1
  Differential Drive Kinematic Model1/2 -> dot/1

== system b6_goto_target/Subsystem1/car_model3 ==
  note: tr=0.6
      | 4T=0.6
      | 一阶系统的动态性能指标为：td=0.69T，tr=2.20T，ts=3T
  vw1 : Inport
  Demux : Demux  Outputs=2
  Differential Drive Kinematic Model1 : robotmobilelib/Differential Drive Kinematic Model  VehicleInputs=Vehicle Speed & Heading Angular Velocity  WheelRadius=0.05  WheelSpeedRange=[-inf inf]  TrackWidth=0.2  InitialState=init_pose_3  SimulateUsing=Interpreted execution
      settings: SourceProductBaseCode=RO
  Simulink顺时针为正 小车逆时针为正 : Gain  Gain=ks
  Transfer Fcn : TransferFcn  Denominator=[0.15 1]
  Transfer Fcn1 : TransferFcn  Denominator=[0.16 1]
  x-y-yaw : Outport
  dot : Outport  Port=2
  wires:
  Simulink顺时针为正 小车逆时针为正/1 -> Transfer Fcn1/1
  Transfer Fcn/1 -> Differential Drive Kinematic Model1/1
  Demux/1 -> Transfer Fcn/1
  Transfer Fcn1/1 -> Differential Drive Kinematic Model1/2
  Demux/2 -> Simulink顺时针为正 小车逆时针为正/1
  vw1/1 -> Demux/1
  Differential Drive Kinematic Model1/1 -> x-y-yaw/1
  Differential Drive Kinematic Model1/2 -> dot/1

== system b6_goto_target/Subsystem1/car_model4 ==
  note: tr=0.6
      | 4T=0.6
      | 一阶系统的动态性能指标为：td=0.69T，tr=2.20T，ts=3T
  vw1 : Inport
  Demux : Demux  Outputs=2
  Differential Drive Kinematic Model1 : robotmobilelib/Differential Drive Kinematic Model  VehicleInputs=Vehicle Speed & Heading Angular Velocity  WheelRadius=0.05  WheelSpeedRange=[-inf inf]  TrackWidth=0.2  InitialState=init_pose_4  SimulateUsing=Interpreted execution
      settings: SourceProductBaseCode=RO
  Simulink顺时针为正 小车逆时针为正 : Gain  Gain=ks
  Transfer Fcn : TransferFcn  Denominator=[0.15 1]
  Transfer Fcn1 : TransferFcn  Denominator=[0.16 1]
  x-y-yaw : Outport
  dot : Outport  Port=2
  wires:
  Simulink顺时针为正 小车逆时针为正/1 -> Transfer Fcn1/1
  Transfer Fcn/1 -> Differential Drive Kinematic Model1/1
  Demux/1 -> Transfer Fcn/1
  Transfer Fcn1/1 -> Differential Drive Kinematic Model1/2
  Demux/2 -> Simulink顺时针为正 小车逆时针为正/1
  vw1/1 -> Demux/1
  Differential Drive Kinematic Model1/1 -> x-y-yaw/1
  Differential Drive Kinematic Model1/2 -> dot/1

== system b6_goto_target/Subsystem1/car_model5 ==
  note: tr=0.6
      | 4T=0.6
      | 一阶系统的动态性能指标为：td=0.69T，tr=2.20T，ts=3T
  vw1 : Inport
  Demux : Demux  Outputs=2
  Differential Drive Kinematic Model1 : robotmobilelib/Differential Drive Kinematic Model  VehicleInputs=Vehicle Speed & Heading Angular Velocity  WheelRadius=0.05  WheelSpeedRange=[-inf inf]  TrackWidth=0.2  InitialState=init_pose_5  SimulateUsing=Interpreted execution
      settings: SourceProductBaseCode=RO
  Simulink顺时针为正 小车逆时针为正 : Gain  Gain=ks
  Transfer Fcn : TransferFcn  Denominator=[0.15 1]
  Transfer Fcn1 : TransferFcn  Denominator=[0.16 1]
  x-y-yaw : Outport
  dot : Outport  Port=2
  wires:
  Simulink顺时针为正 小车逆时针为正/1 -> Transfer Fcn1/1
  Transfer Fcn/1 -> Differential Drive Kinematic Model1/1
  Demux/1 -> Transfer Fcn/1
  Transfer Fcn1/1 -> Differential Drive Kinematic Model1/2
  Demux/2 -> Simulink顺时针为正 小车逆时针为正/1
  vw1/1 -> Demux/1
  Differential Drive Kinematic Model1/1 -> x-y-yaw/1
  Differential Drive Kinematic Model1/2 -> dot/1

== system b6_goto_target/Subsystem1/car_model6 ==
  note: tr=0.6
      | 4T=0.6
      | 一阶系统的动态性能指标为：td=0.69T，tr=2.20T，ts=3T
  vw1 : Inport
  Demux : Demux  Outputs=2
  Differential Drive Kinematic Model1 : robotmobilelib/Differential Drive Kinematic Model  VehicleInputs=Vehicle Speed & Heading Angular Velocity  WheelRadius=0.05  WheelSpeedRange=[-inf inf]  TrackWidth=0.2  InitialState=init_pose_6  SimulateUsing=Interpreted execution
      settings: SourceProductBaseCode=RO
  Simulink顺时针为正 小车逆时针为正 : Gain  Gain=ks
  Transfer Fcn : TransferFcn  Denominator=[0.15 1]
  Transfer Fcn1 : TransferFcn  Denominator=[0.16 1]
  x-y-yaw : Outport
  dot : Outport  Port=2
  wires:
  Simulink顺时针为正 小车逆时针为正/1 -> Transfer Fcn1/1
  Transfer Fcn/1 -> Differential Drive Kinematic Model1/1
  Demux/1 -> Transfer Fcn/1
  Transfer Fcn1/1 -> Differential Drive Kinematic Model1/2
  Demux/2 -> Simulink顺时针为正 小车逆时针为正/1
  vw1/1 -> Demux/1
  Differential Drive Kinematic Model1/1 -> x-y-yaw/1
  Differential Drive Kinematic Model1/2 -> dot/1

== system b6_goto_target/controller1/Subsystem1 ==
  note: Path Following with Obstacle Avoidance in Simulink
  Ranges : Inport
  Angels : Inport  Port=2
  Pose : Inport  Port=3
  WayPoints : Inport  Port=4
  Adjust Velocities to Avoid Obstacles : Subsystem
  Compute Velocity and Heading for Path following : Subsystem
  Constant1 : Constant  Value=scanAngles
  More Info : Subsystem
      settings: OpenFcn=showdemo(bdroot(gcb))
      mask Display: disp('?')
  Outputs : Subsystem
  v : Outport
  w : Outport  Port=2
  CloseToGoal : Outport  Port=3
  wires:
  Outputs/2(w) -> w/1
  Outputs/1(v) -> v/1
  Adjust Velocities to Avoid Obstacles/1(dV) -> Outputs/1(dV)
  Compute Velocity and Heading for Path following/4(CloseToGoal) -> Outputs/5(CloseToGoal), CloseToGoal/1
  WayPoints/1 -> Compute Velocity and Heading for Path following/2(Waypoints)
  Ranges/1 -> Adjust Velocities to Avoid Obstacles/1(Ranges)
  Compute Velocity and Heading for Path following/2(V) -> Adjust Velocities to Avoid Obstacles/4(V), Outputs/3(V)
  Adjust Velocities to Avoid Obstacles/2(dW) -> Outputs/2(dW)
  Pose/1 -> Compute Velocity and Heading for Path following/1(CurrentPose)
  Compute Velocity and Heading for Path following/3(W) -> Adjust Velocities to Avoid Obstacles/5(W), Outputs/4(W)
  Compute Velocity and Heading for Path following/1(TargetDir) -> Adjust Velocities to Avoid Obstacles/3(TargetDir)
  Angels/1 -> Adjust Velocities to Avoid Obstacles/2(Angles)

== system b6_goto_target/controller1/Subsystem2 ==
  note: Path Following with Obstacle Avoidance in Simulink
  Ranges : Inport
  Angels : Inport  Port=2
  Pose : Inport  Port=3
  WayPoints : Inport  Port=4
  Adjust Velocities to Avoid Obstacles : Subsystem
  Compute Velocity and Heading for Path following : Subsystem
  More Info : Subsystem
      settings: OpenFcn=showdemo(bdroot(gcb))
      mask Display: disp('?')
  Outputs : Subsystem
  v : Outport
  w : Outport  Port=2
  CloseToGoal : Outport  Port=3
  wires:
  Angels/1 -> Adjust Velocities to Avoid Obstacles/2(Angles)
  Compute Velocity and Heading for Path following/1(TargetDir) -> Adjust Velocities to Avoid Obstacles/3(TargetDir)
  Compute Velocity and Heading for Path following/3(W) -> Outputs/4(W), Adjust Velocities to Avoid Obstacles/5(W)
  Pose/1 -> Compute Velocity and Heading for Path following/1(CurrentPose)
  Adjust Velocities to Avoid Obstacles/2(dW) -> Outputs/2(dW)
  Compute Velocity and Heading for Path following/2(V) -> Outputs/3(V), Adjust Velocities to Avoid Obstacles/4(V)
  Ranges/1 -> Adjust Velocities to Avoid Obstacles/1(Ranges)
  WayPoints/1 -> Compute Velocity and Heading for Path following/2(Waypoints)
  Compute Velocity and Heading for Path following/4(CloseToGoal) -> CloseToGoal/1, Outputs/5(CloseToGoal)
  Adjust Velocities to Avoid Obstacles/1(dV) -> Outputs/1(dV)
  Outputs/1(v) -> v/1
  Outputs/2(w) -> w/1
